simulink model "refMagtest"  (R2018a)
settings: Solver=FixedStepAuto  StartTime=0  StopTime=10000000  FixedStep=10000  RelTol=1e-3
undefined symbols (not defined in the file or in its folder): Angle, Axis, IAU
libraries: robotcorelib x2, aerolibtransform2 x1, aerolibgravity2 x1
settings Model: Creator=nathan  LastModifiedBy=nathan

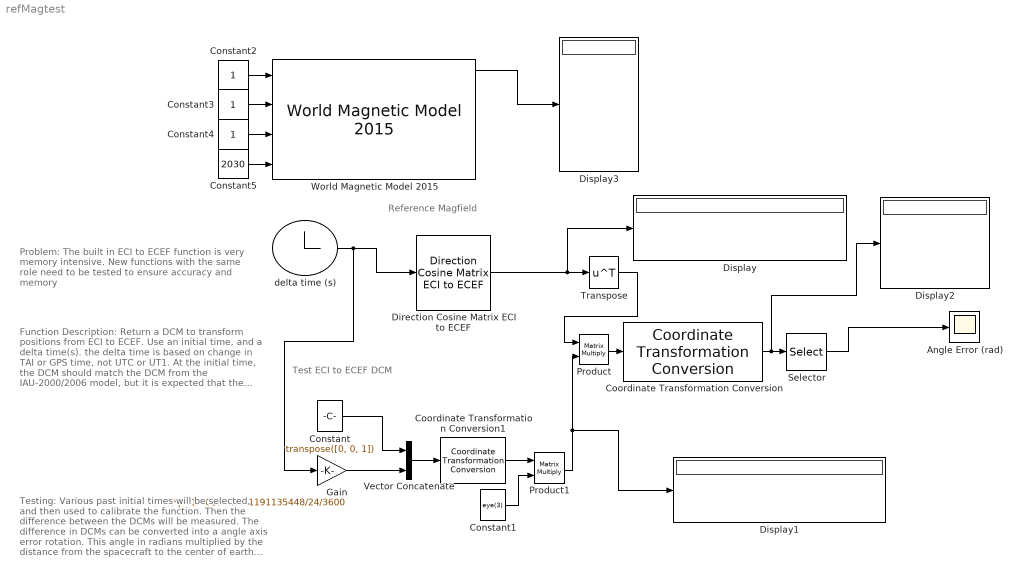
== system refMagtest ==
  note: Reference Magfield
  note: Function Description:
      | Return a DCM to transform positions from ECI to ECEF. Use an initial time, and a delta time(s). the delta time is based on change in TAI or GPS time, not UTC or UT1.
      | At the initial time, the DCM should match the DCM from the IAU-2000/2006 model, but it is expected that the DCMs should slowly drift. This drift must be small enough so that in a few year from initial time, if the DCM is used to transform GPS data in ECEF to ECI, no significant error will be added.
  note: Problem:
      | The built in ECI to ECEF function is very memory intensive. New functions with the same role need to be tested to ensure accuracy and memory
  note: Testing:
      | Various past initial times will be selected, and then used to calibrate the function. Then the difference between the DCMs will be measured. The difference in DCMs can be converted into a angle axis error rotation. This angle in radians multiplied by the distance from the spacecraft to the center of earth will give the maximum offset in distance that the transform added.
  note: Test ECI to ECEF DCM
  Angle Error (rad) : Scope
  Constant : Constant  Value=transpose([0, 0, 1])
  Constant1 : Constant  Value=eye(3)
  Constant2 : Constant
  Constant3 : Constant
  Constant4 : Constant
  Constant5 : Constant  Value=2030
  Coordinate Transformation Conversion : robotcorelib/Coordinate Transformation Conversion  InputRepresentation=Rotation Matrix  InputEulerSequence=ZYX  ShowTrVecInputPort=on  OutputRepresentation=Axis-Angle  OutputEulerSequence=ZYX  ShowTrVecOutputPort=on  SimulateUsing=Interpreted execution
      settings: SourceProductBaseCode=RO
  Coordinate Transformation Conversion1 : robotcorelib/Coordinate Transformation Conversion  InputRepresentation=Axis-Angle  InputEulerSequence=ZYX  ShowTrVecInputPort=on  OutputRepresentation=Rotation Matrix  OutputEulerSequence=ZYX  ShowTrVecOutputPort=on  SimulateUsing=Interpreted execution
      settings: SourceProductBaseCode=RO
  Direction Cosine Matrix ECI to ECEF : aerolibtransform2/Direction Cosine Matrix ECI to ECEF  red=IAU-2000/2006  year=2018  month=January  day=3  hour=0  min=0  sec=0  deltaT=Sec  errorflag=Error  extraparamflag=off
      settings: AttributesFormatString=%<red>  SourceProductName=Aerospace Blockset  SourceProductBaseCode=AE
  Display{,1..3} (4 alike) : Display
  Gain : Gain  Gain=-2*pi*1.00273781191135448/24/3600
  Product : Product  Multiplication=Matrix(*)
  Product1 : Product  Multiplication=Matrix(*)
  Selector : Selector  InputPortWidth=4  IndexOptions=Index vector (dialog)  Indices=[4]  OutputSizes=1
  Transpose : Math  Operator=transpose  SaturateOnIntegerOverflow=on
  Vector Concatenate : Concatenate
  World Magnetic Model 2015 : aerolibgravity2/World Magnetic Model 2015  units=Metric (MKS)  time_in=on  month=January  day=1  year=2015  action=None  h_out=on  dec_out=on  inc_out=on  ti_out=on
      settings: SourceProductName=Aerospace Blockset  SourceProductBaseCode=AE
  delta time (s) : Clock
  wires:
  Transpose/1 -> Product/1
  Coordinate Transformation Conversion/1 -> Display2/1, Selector/1
  Product/1 -> Coordinate Transformation Conversion/1
  Selector/1 -> Angle Error (rad)/1
  Direction Cosine Matrix ECI to ECEF/1 -> Display/1, Transpose/1
  delta time (s)/1 -> Gain/1, Direction Cosine Matrix ECI to ECEF/1
  Vector Concatenate/1 -> Coordinate Transformation Conversion1/1
  Gain/1 -> Vector Concatenate/2
  Constant/1 -> Vector Concatenate/1
  Coordinate Transformation Conversion1/1 -> Product1/1
  Product1/1 -> Display1/1, Product/2
  Constant1/1 -> Product1/2
  Constant2/1 -> World Magnetic Model 2015/1
  Constant3/1 -> World Magnetic Model 2015/2
  Constant4/1 -> World Magnetic Model 2015/3
  Constant5/1 -> World Magnetic Model 2015/4
  World Magnetic Model 2015/1 -> Display3/1
